simulink model "bd_dynamiccomparesims"  (Simulink 4.1.1)
settings: Solver=VariableStepDiscrete  StartTime=0.0  StopTime=inf  FixedStep=1  RelTol=1e-3
undefined symbols (not defined in the file or in its folder): ALTIAHOME
libraries: simulink3 x4
settings Model: LastModifiedBy=abrooker

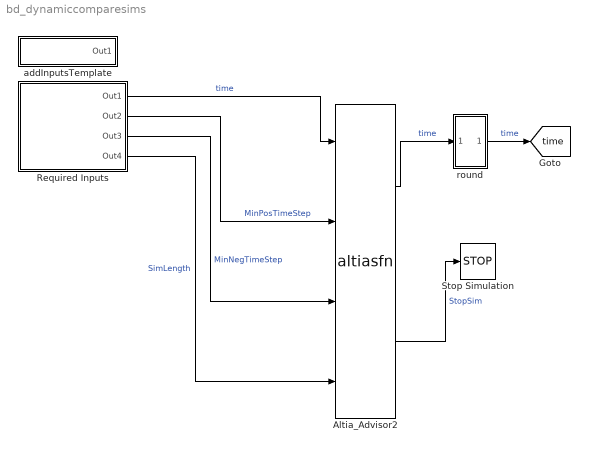
== system bd_dynamiccomparesims ==
  Altia_Advisor2 : S-Function  FunctionName=altiasfn  Parameters=NumAltiaSfnInputs,NumAltiaSfnOutputs,ALTIAHOME  PortCounts=[]  SFunctionModules=libsdde.lib user32.lib  mask{NumAltiaSfnInputs=4, NumAltiaSfnOutputs=2}
      mask prompts: NumAltiaSfnInputs "Inputs to Altia S-Function:"; NumAltiaSfnOutputs "Outputs to Altia S-Function:"
      mask help: This block allows you to connect your signals to an Altia Design file. Specify the number of Inputs and Outputs you would like the Altia block to have (each line connected to the block can only be ONE signal wide ... no muxing into the Altia block).
      mask init:
      | altiahome
      settings: OpenFcn=AltiaClk
      mask Help: The first box is the number of inputs to the Altia S-Function.  The second box is the number of ouputs for the Altia S-Function.
      mask Display: disp('A L T I A')
  Required Inputs : Subsystem
      settings: RTWFcnNameOpts=Auto  RTWFileNameOpts=Auto
      mask Display: disp('Required Inputs');
  Stop Simulation : Stop
  addInputsTemplate : Subsystem  mask{outputVector=, timeVector=}
      mask prompts: outputVector "Output"; timeVector "Time Vector"
      settings: RTWFcnNameOpts=Auto  RTWFileNameOpts=Auto
      mask Display: disp('');
  round : Subsystem  mask{DecPlace=.00001}
      mask prompts: DecPlace "Decimal Place (Example:  .001 rounds 1.2222 to 1.2200)"
      settings: RTWFcnNameOpts=Auto  RTWFileNameOpts=Auto
  tag scope: time=global
  wires:
  Altia_Advisor2/1 -> round/1(In1)  "time"
  Required Inputs/2(Out2) -> Altia_Advisor2/2  "MinPosTimeStep"
  Required Inputs/3(Out3) -> Altia_Advisor2/3  "MinNegTimeStep"
  Required Inputs/4(Out4) -> Altia_Advisor2/4  "SimLength"
  Required Inputs/1(Out1) -> Altia_Advisor2/1  "time"
  round/1(Out1) -> [time]  "time"
  Altia_Advisor2/2 -> Stop Simulation/1  "StopSim"

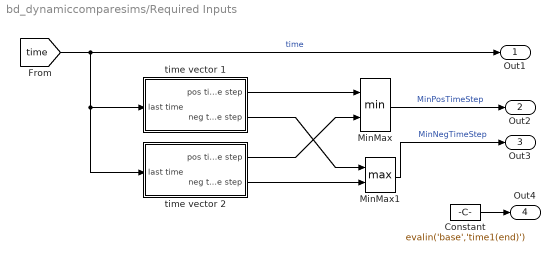
== system bd_dynamiccomparesims/Required Inputs ==
  Constant : Constant  Value=evalin('base','time1(end)')
  MinMax : MinMax  Function=min  Inputs=2
  MinMax1 : MinMax  Function=max  Inputs=2
  time vector 1 : Subsystem  mask{time=evalin('base','time1')}
      mask prompts: time "Time Vector"
      settings: RTWFcnNameOpts=Auto  RTWFileNameOpts=Auto
  time vector 2 : Subsystem  mask{time=evalin('base','time2')}
      mask prompts: time "Time Vector"
      settings: RTWFcnNameOpts=Auto  RTWFileNameOpts=Auto
  Out1 : Outport  Port=1
  Out2 : Outport  Port=2
  Out3 : Outport  Port=3
  Out4 : Outport  Port=4
  wires:
  MinMax/1 -> Out2/1  "MinPosTimeStep"
  MinMax1/1 -> Out3/1  "MinNegTimeStep"
  time vector 1/1(pos time step) -> MinMax/1
  time vector 2/2(neg time step) -> MinMax1/2
  time vector 2/1(pos time step) -> MinMax/2
  time vector 1/2(neg time step) -> MinMax1/1
  [time] -> Out1/1, time vector 1/1(last time), time vector 2/1(last time)  "time"
  Constant/1 -> Out4/1

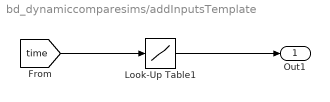
== system bd_dynamiccomparesims/addInputsTemplate ==
  Look-Up Table1 : Lookup  InputValues=timeVector  OutputValues=outputVector
  Out1 : Outport  Port=1
  wires:
  Look-Up Table1/1 -> Out1/1
  [time] -> Look-Up Table1/1

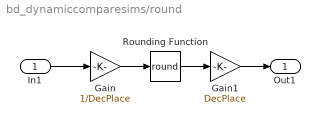
== system bd_dynamiccomparesims/round ==
  In1 : Inport  Port=1  LatchInput=off
  Gain : Gain  Gain=1/DecPlace  Multiplication=Element-wise(K.*u)  SaturateOnIntegerOverflow=on
  Gain1 : Gain  Gain=DecPlace  Multiplication=Element-wise(K.*u)  SaturateOnIntegerOverflow=on
  Rounding Function : Rounding  Operator=round
  Out1 : Outport  Port=1
  wires:
  Rounding Function/1 -> Gain1/1
  Gain/1 -> Rounding Function/1
  In1/1 -> Gain/1
  Gain1/1 -> Out1/1

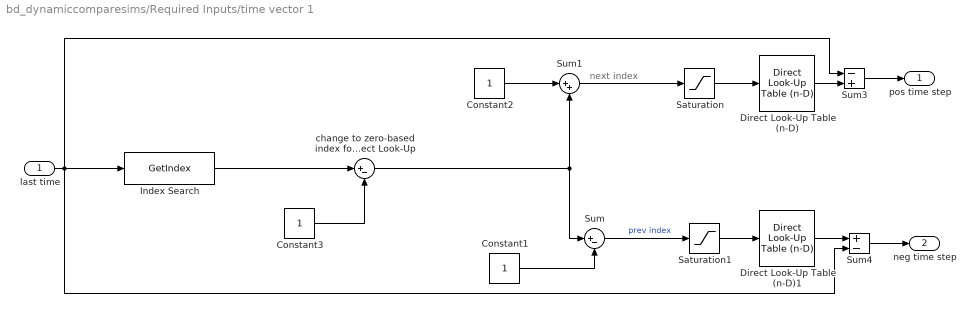
== system bd_dynamiccomparesims/Required Inputs/time vector 1 ==
  note: next index
  last time : Inport  Port=1  LatchInput=off
  Constant1 : Constant  Value=1
  Constant2 : Constant  Value=1
  Constant3 : Constant  Value=1
  Direct Look-Up Table (n-D) : simulink3/Functions & Tables/Direct Look-Up Table (n-D)  maskTabDims=1  explicitNumDims=1  outDims=Element  tabIsInput=off  mxTable=time  clipFlag=None
  Direct Look-Up Table (n-D)1 : simulink3/Functions & Tables/Direct Look-Up Table (n-D)  maskTabDims=1  explicitNumDims=1  outDims=Element  tabIsInput=off  mxTable=time  clipFlag=None
  Index Search : S-Function  FunctionName=GetIndex  Parameters=time  PortCounts=[]  SFunctionModules=''
  Saturation : Saturate  UpperLimit=length(time)  LowerLimit=0  LinearizeAsGain=on
  Saturation1 : Saturate  UpperLimit=length(time)  LowerLimit=0  LinearizeAsGain=on
  Sum : Sum  Inputs=|+-  SaturateOnIntegerOverflow=on
  Sum1 : Sum  Inputs=|++  SaturateOnIntegerOverflow=on
  Sum3 : Sum  Inputs=-+  SaturateOnIntegerOverflow=on
  Sum4 : Sum  Inputs=+-  SaturateOnIntegerOverflow=on
  change to zero-based index for Direct Look-Up : Sum  Inputs=|+-  SaturateOnIntegerOverflow=on
  pos time step : Outport  Port=1
  neg time step : Outport  Port=2
  wires:
  Sum4/1 -> neg time step/1
  Direct Look-Up Table (n-D)1/1 -> Sum4/1
  Direct Look-Up Table (n-D)/1 -> Sum3/2
  Sum3/1 -> pos time step/1
  last time/1 -> Index Search/1, Sum3/1, Sum4/2
  Saturation1/1 -> Direct Look-Up Table (n-D)1/1
  Saturation/1 -> Direct Look-Up Table (n-D)/1
  Sum1/1 -> Saturation/1
  Constant2/1 -> Sum1/1
  Constant1/1 -> Sum/2
  Sum/1 -> Saturation1/1  "prev index"
  Index Search/1 -> change to zero-based index for Direct Look-Up/1
  change to zero-based index for Direct Look-Up/1 -> Sum1/2, Sum/1
  Constant3/1 -> change to zero-based index for Direct Look-Up/2

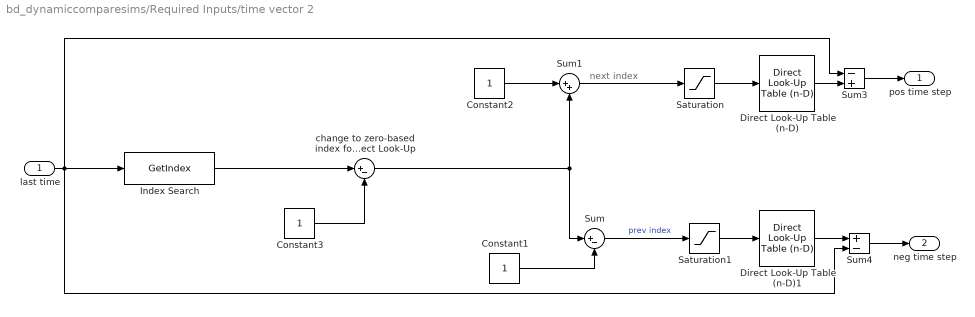
== system bd_dynamiccomparesims/Required Inputs/time vector 2 ==
  note: next index
  last time : Inport  Port=1  LatchInput=off
  Constant1 : Constant  Value=1
  Constant2 : Constant  Value=1
  Constant3 : Constant  Value=1
  Direct Look-Up Table (n-D) : simulink3/Functions & Tables/Direct Look-Up Table (n-D)  maskTabDims=1  explicitNumDims=1  outDims=Element  tabIsInput=off  mxTable=time  clipFlag=None
  Direct Look-Up Table (n-D)1 : simulink3/Functions & Tables/Direct Look-Up Table (n-D)  maskTabDims=1  explicitNumDims=1  outDims=Element  tabIsInput=off  mxTable=time  clipFlag=None
  Index Search : S-Function  FunctionName=GetIndex  Parameters=time  PortCounts=[]  SFunctionModules=''
  Saturation : Saturate  UpperLimit=length(time)  LowerLimit=0  LinearizeAsGain=on
  Saturation1 : Saturate  UpperLimit=length(time)  LowerLimit=0  LinearizeAsGain=on
  Sum : Sum  Inputs=|+-  SaturateOnIntegerOverflow=on
  Sum1 : Sum  Inputs=|++  SaturateOnIntegerOverflow=on
  Sum3 : Sum  Inputs=-+  SaturateOnIntegerOverflow=on
  Sum4 : Sum  Inputs=+-  SaturateOnIntegerOverflow=on
  change to zero-based index for Direct Look-Up : Sum  Inputs=|+-  SaturateOnIntegerOverflow=on
  pos time step : Outport  Port=1
  neg time step : Outport  Port=2
  wires:
  Constant3/1 -> change to zero-based index for Direct Look-Up/2
  change to zero-based index for Direct Look-Up/1 -> Sum/1, Sum1/2
  Index Search/1 -> change to zero-based index for Direct Look-Up/1
  Sum/1 -> Saturation1/1  "prev index"
  Constant1/1 -> Sum/2
  Constant2/1 -> Sum1/1
  Sum1/1 -> Saturation/1
  Saturation/1 -> Direct Look-Up Table (n-D)/1
  Saturation1/1 -> Direct Look-Up Table (n-D)1/1
  last time/1 -> Sum4/2, Sum3/1, Index Search/1
  Sum3/1 -> pos time step/1
  Direct Look-Up Table (n-D)/1 -> Sum3/2
  Direct Look-Up Table (n-D)1/1 -> Sum4/1
  Sum4/1 -> neg time step/1
